simulink model "MPC_VS_FOCCopy_ST_Psim12"  (R2021a)
settings: Solver=VariableStepAuto  StartTime=0.0  StopTime=0.3  FixedStep=1/150000  MaxStep=1e-6
libraries: spsMosfetLib x12, simulink x7, pid_lib x3, spsFirstOrderFilterLib x2, spsPermanentMagnetSynchronousMachineLib x2, spsCurrentMeasurementLib x2, spsDCVoltageSourceLib x2, spsThreePhaseVIMeasurementLib x2, spsabctodq0Lib x2, spsSVPWMGenerator2LevelLib x1, spsdq0toAlphaBetaZeroLib x1, spspowerguiLib x1
settings Model: Creator=Hassan Alam  LastModifiedBy=zero
settings SolverCC: ZeroCrossAlgorithm=Adaptive
settings DebuggingCC: MaskedZcDiagnostic=none  IgnoredZcDiagnostic=none  SFMachineParentedDataDiag=warning  ArithmeticOperatorsInVariantConditions=warning
settings SFSimCC: CustomCodeUndefinedFunction=UseInterfaceOnly

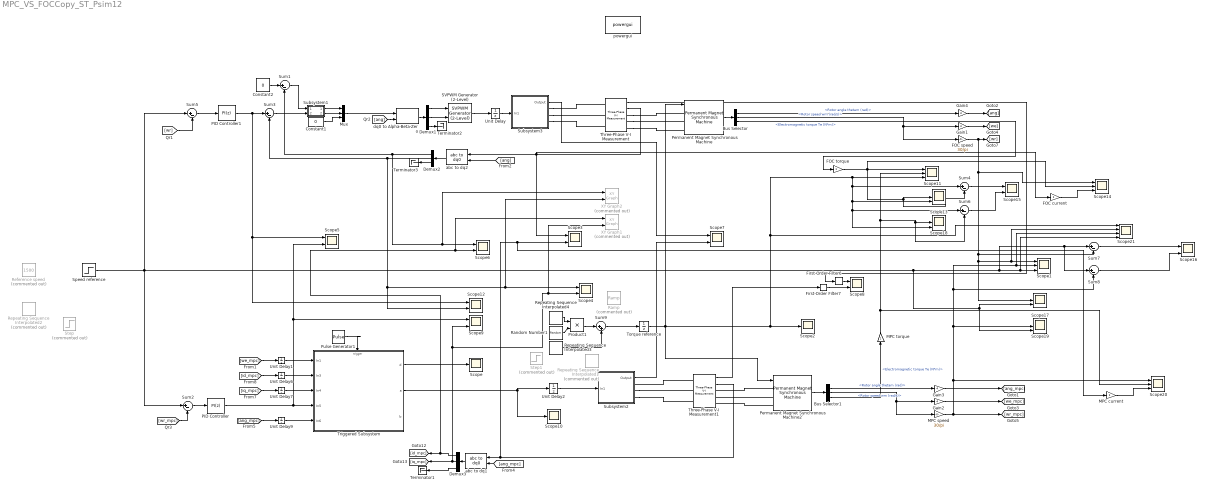
== system MPC_VS_FOCCopy_ST_Psim12 ==
  Bus Selector : BusSelector  OutputSignals=Rotor angle thetam (rad),Rotor speed wm (rad/s),Electromagnetic torque Te (N*m)
  Bus Selector1 : BusSelector  OutputSignals=Rotor angle thetam (rad),Rotor speed wm (rad/s),Electromagnetic torque Te (N*m)
  Constant1 : Constant  Value=0
  Constant2 : Constant  Value=0
  Demux1 : Demux  Outputs=3
  Demux2 : Demux  Outputs=3
  Demux3 : Demux  Outputs=3
  FOC current : Gain
  FOC speed : Gain  Gain=30/pi
  FOC torque : Gain
  First-Order Filter6 : spsFirstOrderFilterLib/First-Order Filter  FilterType=Lowpass  Tc=1e-3  Ts=0  Initialize=on  Vac_Init=[0, 0, 60]  Vdc_Init=0  PlotResponse=off  FreqRange="[0,  200,  1]"
  First-Order Filter7 : spsFirstOrderFilterLib/First-Order Filter  FilterType=Lowpass  Tc=1e-3  Ts=0  Initialize=on  Vac_Init=[0, 0, 60]  Vdc_Init=0  PlotResponse=off  FreqRange="[0,  200,  1]"
  Gain{1..4} (4 alike) : Gain  Gain=4
  MPC current : Gain
  MPC speed : Gain  Gain=30/pi
  MPC torque : Gain
  Mux : Mux  Inputs=3
  PID Controller : pid_lib/PID Controller  Controller=PI  Form=Parallel  TimeDomain=Discrete-time  UseExternalTs=off  SampleTime=1/4000  IntegratorMethod=Forward Euler  FilterMethod=Forward Euler  ControllerParametersSource=internal  P=0.02  I=20  D=0  UseFilter=on  N=100  TunerSelectOption=Transfer Function Based (PID Tuner App)  InitialConditionSource=internal  InitialConditionForIntegrator=0  InitialConditionForFilter=0  DifferentiatorICPrevScaledInput=0  ExternalReset=none  TrackingMode=off  Kt=1  LimitOutput=on  SatLimitsSource=internal  UpperSaturationLimit=3  LowerSaturationLimit=-3  LinearizeAsGain=on  AntiWindupMode=clamping  Kb=1  POutMin=[]  POutMax=[]  IOutMin=[]  IOutMax=[]  DOutMin=[]  DOutMax=[]  NOutMin=[]  NOutMax=[]  SumOutMin=[]  SumOutMax=[]  SaturationOutMin=[]  SaturationOutMax=[]  PParamMin=[]  PParamMax=[]  IParamMin=[]  IParamMax=[]  DParamMin=[]  DParamMax=[]  NParamMin=[]  NParamMax=[]  KbParamMin=[]  KbParamMax=[]  KtParamMin=[]  KtParamMax=[]  KbOutMin=[]  KbOutMax=[]  KtOutMin=[]  KtOutMax=[]  IntegratorOutMin=[]  IntegratorOutMax=[]  FilterOutMin=[]  FilterOutMax=[]  SumI1OutMin=[]  SumI1OutMax=[]  SumI2OutMin=[]  SumI2OutMax=[]  SumI3OutMin=[]  SumI3OutMax=[]  SumI4OutMin=[]  SumI4OutMax=[]  SumDOutMin=[]  SumDOutMax=[]  DifferentiatorOutMin=[]  DifferentiatorOutMax=[]  FilterDiffOutCoefMin=[]  FilterDiffOutCoefMax=[]  ReciprocalOutMin=[]  ReciprocalOutMax=[]  SumDenOutMin=[]  SumDenOutMax=[]  SumNumOutMin=[]  SumNumOutMax=[]  DivideOutMin=[]  DivideOutMax=[]  UdiffTsProdOutMin=[]  UdiffTsProdOutMax=[]  NTsProdOutMin=[]  NTsProdOutMax=[]  UintegralTsProdOutMin=[]  UintegralTsProdOutMax=[]  UngainTsProdOutMin=[]  UngainTsProdOutMax=[]  IntegratorContinuousStateAttributes=''  IntegratorStateMustResolveToSignalObject=off  IntegratorRTWStateStorageClass=Auto  FilterContinuousStateAttributes=''  FilterStateMustResolveToSignalObject=off  FilterRTWStateStorageClass=Auto  ParallelPVariant=InternalParameters  IdealPVariant=Disabled  IVariant=InternalParameters  DVariant=Disabled  IntegratorVariant=Discrete  SatVariant=Enabled  AWVariant=DiscClampingParallel  PCopyVariant=Disabled  TRVariant=Disabled  FdbkBlocksVariant=Forward  IdealPFdbkVariant=Disabled  SatFdbkVariant=Disabled  DerivativeFilterVariant=Disabled  NVariant=Disabled  NCopyVariant=Disabled_SignalSpec  FilterICVariant=Disabled  IntegratorICVariant=InternalICs  ExternalResetVariant=Disabled  TRSumVariant=Passthrough  SumFdbkVariant=Disabled  SumVariant=Sum_PI  TsampFilterVariant=InternalTs  TsampNgainVariant=Passthrough  TsampIntegralVariant=Passthrough  ExternalSaturationOutDataTypeStr=Inherit: Same as second input
  PID Controller1 : pid_lib/PID Controller  Controller=PI  Form=Parallel  TimeDomain=Discrete-time  UseExternalTs=off  SampleTime=1/4000  IntegratorMethod=Forward Euler  FilterMethod=Forward Euler  ControllerParametersSource=internal  P=0.02  I=20  D=0  UseFilter=on  N=100  TunerSelectOption=Transfer Function Based (PID Tuner App)  InitialConditionSource=internal  InitialConditionForIntegrator=0  InitialConditionForFilter=0  DifferentiatorICPrevScaledInput=0  ExternalReset=none  TrackingMode=off  Kt=1  LimitOutput=on  SatLimitsSource=internal  UpperSaturationLimit=3  LowerSaturationLimit=-3  LinearizeAsGain=on  AntiWindupMode=clamping  Kb=1  POutMin=[]  POutMax=[]  IOutMin=[]  IOutMax=[]  DOutMin=[]  DOutMax=[]  NOutMin=[]  NOutMax=[]  SumOutMin=[]  SumOutMax=[]  SaturationOutMin=[]  SaturationOutMax=[]  PParamMin=[]  PParamMax=[]  IParamMin=[]  IParamMax=[]  DParamMin=[]  DParamMax=[]  NParamMin=[]  NParamMax=[]  KbParamMin=[]  KbParamMax=[]  KtParamMin=[]  KtParamMax=[]  KbOutMin=[]  KbOutMax=[]  KtOutMin=[]  KtOutMax=[]  IntegratorOutMin=[]  IntegratorOutMax=[]  FilterOutMin=[]  FilterOutMax=[]  SumI1OutMin=[]  SumI1OutMax=[]  SumI2OutMin=[]  SumI2OutMax=[]  SumI3OutMin=[]  SumI3OutMax=[]  SumI4OutMin=[]  SumI4OutMax=[]  SumDOutMin=[]  SumDOutMax=[]  DifferentiatorOutMin=[]  DifferentiatorOutMax=[]  FilterDiffOutCoefMin=[]  FilterDiffOutCoefMax=[]  ReciprocalOutMin=[]  ReciprocalOutMax=[]  SumDenOutMin=[]  SumDenOutMax=[]  SumNumOutMin=[]  SumNumOutMax=[]  DivideOutMin=[]  DivideOutMax=[]  UdiffTsProdOutMin=[]  UdiffTsProdOutMax=[]  NTsProdOutMin=[]  NTsProdOutMax=[]  UintegralTsProdOutMin=[]  UintegralTsProdOutMax=[]  UngainTsProdOutMin=[]  UngainTsProdOutMax=[]  IntegratorContinuousStateAttributes=''  IntegratorStateMustResolveToSignalObject=off  IntegratorRTWStateStorageClass=Auto  FilterContinuousStateAttributes=''  FilterStateMustResolveToSignalObject=off  FilterRTWStateStorageClass=Auto  ParallelPVariant=InternalParameters  IdealPVariant=Disabled  IVariant=InternalParameters  DVariant=Disabled  IntegratorVariant=Discrete  SatVariant=Enabled  AWVariant=DiscClampingParallel  PCopyVariant=Disabled  TRVariant=Disabled  FdbkBlocksVariant=Forward  IdealPFdbkVariant=Disabled  SatFdbkVariant=Disabled  DerivativeFilterVariant=Disabled  NVariant=Disabled  NCopyVariant=Disabled_SignalSpec  FilterICVariant=Disabled  IntegratorICVariant=InternalICs  ExternalResetVariant=Disabled  TRSumVariant=Passthrough  SumFdbkVariant=Disabled  SumVariant=Sum_PI  TsampFilterVariant=InternalTs  TsampNgainVariant=Passthrough  TsampIntegralVariant=Passthrough  ExternalSaturationOutDataTypeStr=Inherit: Same as second input
  Permanent Magnet Synchronous Machine : spsPermanentMagnetSynchronousMachineLib/Permanent Magnet Synchronous Machine  NbPhases=3  FluxDistribution=Sinusoidal  RotorType=Round  MechanicalLoad=Torque Tm  PresetModel=No  ShowDetailedParameters=on  MeasurementBus=off  Resistance=0.75  Inductance=8.5e-3  dqInductances=[8.5e-3,8.5e-3]  La=0.0004  MachineConstant=Flux linkage established by magnets (V.s)  Flux=0.00666  VoltageCst=4.832  TorqueCst=0.03996  Flat=120  Mechanical=[2.66e-6 1.33e-6 4 0]  PolePairs=4  InitialConditions=[0,0, 0,0]  InitialConditions5ph=[0 0 0 0 0 0]  RefAngle=90 degrees behind phase A axis (modified Park)  IterativeDiscreteModel=Trapezoidal non iterative  TsBlock=-1  TsPowergui=0
  Permanent Magnet Synchronous Machine2 : spsPermanentMagnetSynchronousMachineLib/Permanent Magnet Synchronous Machine  NbPhases=3  FluxDistribution=Sinusoidal  RotorType=Round  MechanicalLoad=Torque Tm  PresetModel=No  ShowDetailedParameters=on  MeasurementBus=off  Resistance=0.75  Inductance=8.5e-3  dqInductances=[8.5e-3,8.5e-3]  La=0.0004  MachineConstant=Flux linkage established by magnets (V.s)  Flux=0.00666  VoltageCst=4.832  TorqueCst=0.03996  Flat=120  Mechanical=[2.66e-6 1.33e-6 4 0]  PolePairs=4  InitialConditions=[0,0, 0,0]  InitialConditions5ph=[0 0 0 0 0 0]  RefAngle=90 degrees behind phase A axis (modified Park)  IterativeDiscreteModel=Trapezoidal non iterative  TsBlock=-1  TsPowergui=0
  Product1 : Product
  Pulse Generator1 : DiscretePulseGenerator  PulseType=Time based  Period=1/40000  PulseWidth=5
  Ramp : simulink/Sources/Ramp  Commented=on  slope=1  start=0  InitialOutput=0
  Random Number1 : RandomNumber  Seed=123  SampleTime=1e-4*2
  Reference speed : Constant  Commented=on  Value=1500
  Repeating Sequence Interpolated1 : simulink/Sources/Repeating Sequence Interpolated  Commented=on  OutValues=[0 0 0.1 0.1 -0.1 -0.1].'  TimeValues=[0 0.1 0.10001 0.3 0.30001 0.4].'  LookUpMeth=Interpolation-Use End Values  tsamp=1e-6  OutMin=[]  OutMax=[]  OutDataTypeStr=double  OutputDataTypeScalingMode=double  OutDataType=fixdt(0,8)  OutScaling=2^-10
  Repeating Sequence Interpolated2 : simulink/Sources/Repeating Sequence Interpolated  Commented=on  OutValues=[1500 1500 800 800 1200 1200 500 500 1000 1000 1500 1500 0].'  TimeValues=[0 0.0229 0.023 0.0499 0.05 0.095 0.10 0.159 0.16 0.20 0.22 0.27 0.3].'/0.333  LookUpMeth=Interpolation-Use End Values  tsamp=1e-6  OutMin=[]  OutMax=[]  OutDataTypeStr=double  OutputDataTypeScalingMode=double  OutDataType=fixdt(0,8)  OutScaling=2^-10
  Repeating Sequence Interpolated3 : simulink/Sources/Repeating Sequence Interpolated  OutValues=[0 0.05 0.1 0.1 0.1 0.125 0.125 0.05 0].'*0.7  TimeValues=[0 0.01 0.02 0.05 0.15 0.16 0.25 0.27 0.3].'  LookUpMeth=Interpolation-Use End Values  tsamp=1e-6  OutMin=[]  OutMax=[]  OutDataTypeStr=double  OutputDataTypeScalingMode=double  OutDataType=fixdt(0,8)  OutScaling=2^-10
  Repeating Sequence Interpolated4 : simulink/Sources/Repeating Sequence Interpolated  OutValues=[0 0.008 0.015 0.015 0.015 0.02 0.02 0.008 0].'  TimeValues=[0 0.01 0.02 0.05 0.15 0.16 0.25 0.27 0.3].'  LookUpMeth=Interpolation-Use End Values  tsamp=1e-6  OutMin=[]  OutMax=[]  OutDataTypeStr=double  OutputDataTypeScalingMode=double  OutDataType=fixdt(0,8)  OutScaling=2^-10
  SVPWM Generator (2-Level) : spsSVPWMGenerator2LevelLib/SVPWM Generator (2-Level)  InputType=alpha-beta components  SwitchingPattern=Pattern #1  Fc=40000  ParUref=[0.8 -30 50]  Ts=0
      settings: SourceProductBaseCode=PS
  Scope : Scope
  Scope{1,11,13..14,17..20} (8 alike) : Scope  NumInputPorts=3
  Scope10 : Scope
  Scope{3..9,12,15..16} (10 alike) : Scope  NumInputPorts=2
  Scope2 : Scope
  Scope21 : Scope  NumInputPorts=4
  Speed reference : Step  Time=0.2  Before=1500  After=1500  SampleTime=0
  Step : Step  Commented=on  Time=0  After=800  SampleTime=0
  Step1 : Step  Commented=on  Time=0.1  After=0.1  SampleTime=0
  Subsystem1 : Subsystem
  Subsystem2 : Subsystem
  Subsystem3 : Subsystem
  Sum{1..8} (8 alike) : Sum  Inputs=|+-
  Sum9 : Sum  Inputs=|++
  Terminator1 : Terminator
  Terminator2 : Terminator
  Terminator3 : Terminator
  Three-Phase V-I Measurement : spsThreePhaseVIMeasurementLib/Three-Phase V-I Measurement  VoltageMeasurement=phase-to-phase  SetLabelV=off  LabelV=Vabc  Vpu=off  VpuLL=off  CurrentMeasurement=yes  SetLabelI=off  LabelI=Iabc  Ipu=off  Pbase=100e6  Vbase=500e3  OutputType=Complex  PhasorSimulation=off  PSBequivalent=0
  Three-Phase V-I Measurement1 : spsThreePhaseVIMeasurementLib/Three-Phase V-I Measurement  VoltageMeasurement=phase-to-phase  SetLabelV=off  LabelV=Vabc  Vpu=off  VpuLL=off  CurrentMeasurement=yes  SetLabelI=off  LabelI=Iabc  Ipu=off  Pbase=100e6  Vbase=500e3  OutputType=Complex  PhasorSimulation=off  PSBequivalent=0
  Torque reference : UnitDelay  SampleTime=1e-6  HasFrameUpgradeWarning=on
  Triggered Subsystem : Subsystem  TreatAsAtomicUnit=on
  Unit Delay : UnitDelay  SampleTime=1e-6  HasFrameUpgradeWarning=on
  Unit Delay{1,6..7,9} (4 alike) : UnitDelay  SampleTime=-1  HasFrameUpgradeWarning=on
  Unit Delay2 : UnitDelay  SampleTime=1e-6  HasFrameUpgradeWarning=on
  XY Graph1 : simulink/Sinks/XY Graph  Commented=on  xmin=-5  xmax=5  ymin=-5  ymax=5  st=-1
  XY Graph2 : simulink/Sinks/XY Graph  Commented=on  xmin=-5  xmax=5  ymin=-5  ymax=5  st=-1
  abc to dq1 : spsabctodq0Lib/abc to dq0  Alignment=90 degrees behind phase A axis
  abc to dq2 : spsabctodq0Lib/abc to dq0  Alignment=90 degrees behind phase A axis
  dq0 to Alpha-Beta-Zero : spsdq0toAlphaBetaZeroLib/dq0 to Alpha-Beta-Zero  Alignment=90 degrees behind phase A axis
      settings: SourceProductBaseCode=PS
  powergui : spspowerguiLib/powergui  Priority=1  SimulationMode=Continuous  SampleTime=1e-6  frequency=60  Iterations=50  frequencyindice=0  Pbase=100e6  ErrMax=1e-4  UnitsV=kV  UnitsW=MW  buscounter=0  FunctionMessages=off  echomessages=off  EnableUseOfTLC=off  CurrentSourceSwitches=off  DisableSnubberDevices=off  DisableRonSwitches=off  DisableVfSwitches=off  DisplayEquations=off  AutomaticDiscreteSolvers=off  SolverType=Tustin/Backward Euler (TBE)  Interpol=off  ExternalGateDelay=off  methode=off  Ts=100  x0status=blocks  SPID=on  SwTol=0  HookPort=off  NonlinearTolerance=1e-4  nMaxIteration=100  ContinueOnMaxIteration=off  RestoreLinks=warning  ResistiveCurrentMeasurement=off  Frange=[0:2:500]  Ylog=off  Xlog=on  ShowGrid=off  save=off  variable=ZData  structure=0  ZoomFFT=off  StartTime=0.0  cycles=1  DisplayStyle=1  fundamental=60  FreqAxis=off  MaxFrequency=1000  frequencyindicesteady=1  RmsSteady=1  display=off
  wires:
  [wr] -> Sum5/2
  Unit Delay7/1 -> Triggered Subsystem/3(In4)
  [we_mpc] -> Unit Delay1/1
  [ang_mpc] -> Unit Delay9/1
  [iq_mpc] -> Unit Delay7/1
  PID Controller/1 -> Scope9/1, Scope5/2, Triggered Subsystem/4(In5)
  Unit Delay1/1 -> Triggered Subsystem/1(In1)
  [id_mpc] -> Unit Delay6/1
  Unit Delay6/1 -> Triggered Subsystem/2(In3)
  Unit Delay9/1 -> Triggered Subsystem/5(In6)
  Pulse Generator1/1 -> Triggered Subsystem/Trigger
  Constant2/1 -> Sum1/1
  dq0 to Alpha-Beta-Zero/1 -> Demux1/1
  Demux1/2 -> SVPWM Generator (2-Level)/2
  Demux1/1 -> SVPWM Generator (2-Level)/1
  Demux1/3 -> Terminator2/1
  [ang] -> dq0 to Alpha-Beta-Zero/2
  Constant1/1 -> Mux/3
  abc to dq2/1 -> Demux2/1
  Gain4/1 -> [ang]
  Gain1/1 -> [we]
  [ang] -> abc to dq2/2
  Demux2/3 -> Terminator3/1
  Demux3/3 -> Terminator1/1
  [ang_mpc] -> abc to dq1/2
  abc to dq1/1 -> Demux3/1
  Three-Phase V-I Measurement1/2 -> MPC current/1, Scope3/2, abc to dq1/1
  Three-Phase V-I Measurement/2 -> Scope3/1, FOC current/1, abc to dq2/1
  Demux2/2 -> Sum3/2, Scope12/2, XY Graph2/2, Scope4/1
  Demux3/2 -> [iq_mpc], Scope9/2, XY Graph1/2, Scope4/2
  Demux3/1 -> XY Graph1/1, Scope6/2, [id_mpc]
  Demux2/1 -> XY Graph2/1, Scope6/1, Sum1/2
  First-Order Filter7/1 -> Scope8/2
  First-Order Filter6/1 -> Scope8/1
  Three-Phase V-I Measurement1/1 -> First-Order Filter7/1
  Three-Phase V-I Measurement/1 -> First-Order Filter6/1
  Sum5/1 -> PID Controller1/1
  Speed reference/1 -> Sum5/1, Scope19/3, Scope17/3, Sum8/1, Sum7/1, Scope21/4, Scope1/3, Sum2/1
  [wr_mpc] -> Sum2/2
  Sum1/1 -> Subsystem1/1(In1)
  Sum3/1 -> Subsystem1/2(In2)
  Subsystem1/1(Out1) -> Mux/1
  Subsystem1/2(Out2) -> Mux/2
  Sum2/1 -> PID Controller/1
  Torque reference/1 -> Scope21/1, Sum4/1, Scope13/3, Scope18/3, Sum6/1, Scope11/3, Scope2/1, Permanent Magnet Synchronous Machine2/1, Permanent Magnet Synchronous Machine/1
  Subsystem3/1(Output) -> Scope7/1
  PID Controller1/1 -> Scope12/1, Scope5/1, Sum3/1
  Mux/1 -> dq0 to Alpha-Beta-Zero/1
  SVPWM Generator (2-Level)/1 -> Unit Delay/1
  Unit Delay/1 -> Subsystem3/1(In1)
  Permanent Magnet Synchronous Machine/1 -> Bus Selector/1
  Bus Selector/1 -> Gain4/1  "<Rotor angle thetam (rad)>"
  Bus Selector/2 -> FOC speed/1, Gain1/1  "<Rotor speed wm (rad/s)>"
  Bus Selector1/2 -> Gain2/1, MPC speed/1  "<Rotor speed wm (rad/s)>"
  Bus Selector1/1 -> Gain3/1  "<Rotor angle thetam (rad)>"
  Permanent Magnet Synchronous Machine2/1 -> Bus Selector1/1
  Gain2/1 -> [we_mpc]
  Gain3/1 -> [ang_mpc]
  Unit Delay2/1 -> Subsystem2/1(In1)
  Subsystem2/1(Output) -> Scope7/2
  Bus Selector/3 -> FOC torque/1  "<Electromagnetic torque Te (N*m)>"
  Bus Selector1/3 -> MPC torque/1  "<Electromagnetic torque Te (N*m)>"
  MPC torque/1 -> Scope20/2, Scope18/2, Sum6/2, Scope11/2
  FOC torque/1 -> Scope14/2, Sum4/2, Scope13/2, Scope11/1
  Sum6/1 -> Scope15/2
  Sum4/1 -> Scope15/1
  Sum7/1 -> Scope16/1
  Sum8/1 -> Scope16/2
  FOC speed/1 -> Scope14/1, Scope17/2, Scope21/2, Scope1/1, Sum7/2, [wr]
  MPC speed/1 -> Scope19/2, Sum8/2, Scope21/3, Scope1/2, Scope20/1, [wr_mpc]
  Random Number1/1 -> Product1/2
  Repeating Sequence Interpolated4/1 -> Product1/1
  Repeating Sequence Interpolated3/1 -> Sum9/2
  Product1/1 -> Sum9/1
  Triggered Subsystem/2(a) -> Scope10/1, Unit Delay2/1
  Triggered Subsystem/1(d) -> Scope/1
  FOC current/1 -> Scope14/3
  MPC current/1 -> Scope20/3
  Sum9/1 -> Torque reference/1
  connections:
  Subsystem3/RConn1 -- Three-Phase V-I Measurement/LConn1
  Subsystem3/RConn2 -- Three-Phase V-I Measurement/LConn2
  Subsystem3/RConn3 -- Three-Phase V-I Measurement/LConn3
  Three-Phase V-I Measurement/RConn1 -- Permanent Magnet Synchronous Machine/LConn1
  Three-Phase V-I Measurement/RConn2 -- Permanent Magnet Synchronous Machine/LConn2
  Three-Phase V-I Measurement/RConn3 -- Permanent Magnet Synchronous Machine/LConn3
  Permanent Magnet Synchronous Machine2/LConn3 -- Three-Phase V-I Measurement1/RConn3
  Permanent Magnet Synchronous Machine2/LConn1 -- Three-Phase V-I Measurement1/RConn1
  Subsystem2/RConn2 -- Three-Phase V-I Measurement1/LConn2
  Subsystem2/RConn3 -- Three-Phase V-I Measurement1/LConn3
  Three-Phase V-I Measurement1/LConn1 -- Subsystem2/RConn1
  Permanent Magnet Synchronous Machine2/LConn2 -- Three-Phase V-I Measurement1/RConn2

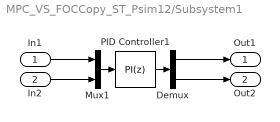
== system MPC_VS_FOCCopy_ST_Psim12/Subsystem1 ==
  In1 : Inport
  In2 : Inport  Port=2
  Demux : Demux  Outputs=2
  Mux1 : Mux  Inputs=2
  PID Controller1 : pid_lib/PID Controller  Controller=PI  Form=Parallel  TimeDomain=Discrete-time  UseExternalTs=off  SampleTime=1/40000  IntegratorMethod=Forward Euler  FilterMethod=Forward Euler  ControllerParametersSource=internal  P=1  I=800  D=0  UseFilter=on  N=100  TunerSelectOption=Transfer Function Based (PID Tuner App)  InitialConditionSource=internal  InitialConditionForIntegrator=0  InitialConditionForFilter=0  DifferentiatorICPrevScaledInput=0  ExternalReset=none  TrackingMode=off  Kt=1  LimitOutput=off  SatLimitsSource=internal  UpperSaturationLimit=3  LowerSaturationLimit=-3  LinearizeAsGain=on  AntiWindupMode=clamping  Kb=1  POutMin=[]  POutMax=[]  IOutMin=[]  IOutMax=[]  DOutMin=[]  DOutMax=[]  NOutMin=[]  NOutMax=[]  SumOutMin=[]  SumOutMax=[]  SaturationOutMin=[]  SaturationOutMax=[]  PParamMin=[]  PParamMax=[]  IParamMin=[]  IParamMax=[]  DParamMin=[]  DParamMax=[]  NParamMin=[]  NParamMax=[]  KbParamMin=[]  KbParamMax=[]  KtParamMin=[]  KtParamMax=[]  KbOutMin=[]  KbOutMax=[]  KtOutMin=[]  KtOutMax=[]  IntegratorOutMin=[]  IntegratorOutMax=[]  FilterOutMin=[]  FilterOutMax=[]  SumI1OutMin=[]  SumI1OutMax=[]  SumI2OutMin=[]  SumI2OutMax=[]  SumI3OutMin=[]  SumI3OutMax=[]  SumI4OutMin=[]  SumI4OutMax=[]  SumDOutMin=[]  SumDOutMax=[]  DifferentiatorOutMin=[]  DifferentiatorOutMax=[]  FilterDiffOutCoefMin=[]  FilterDiffOutCoefMax=[]  ReciprocalOutMin=[]  ReciprocalOutMax=[]  SumDenOutMin=[]  SumDenOutMax=[]  SumNumOutMin=[]  SumNumOutMax=[]  DivideOutMin=[]  DivideOutMax=[]  UdiffTsProdOutMin=[]  UdiffTsProdOutMax=[]  NTsProdOutMin=[]  NTsProdOutMax=[]  UintegralTsProdOutMin=[]  UintegralTsProdOutMax=[]  UngainTsProdOutMin=[]  UngainTsProdOutMax=[]  IntegratorContinuousStateAttributes=''  IntegratorStateMustResolveToSignalObject=off  IntegratorRTWStateStorageClass=Auto  FilterContinuousStateAttributes=''  FilterStateMustResolveToSignalObject=off  FilterRTWStateStorageClass=Auto  ParallelPVariant=InternalParameters  IdealPVariant=Disabled  IVariant=InternalParameters  DVariant=Disabled  IntegratorVariant=Discrete  SatVariant=Disabled  AWVariant=Passthrough  PCopyVariant=Disabled  TRVariant=Disabled  FdbkBlocksVariant=Forward  IdealPFdbkVariant=Disabled  SatFdbkVariant=Disabled  DerivativeFilterVariant=Disabled  NVariant=Disabled  NCopyVariant=Disabled_SignalSpec  FilterICVariant=Disabled  IntegratorICVariant=InternalICs  ExternalResetVariant=Disabled  TRSumVariant=Passthrough  SumFdbkVariant=Disabled  SumVariant=Sum_PI  TsampFilterVariant=InternalTs  TsampNgainVariant=Passthrough  TsampIntegralVariant=Passthrough  ExternalSaturationOutDataTypeStr=Inherit: Same as second input
  Out1 : Outport
  Out2 : Outport  Port=2
  wires:
  In1/1 -> Mux1/1
  Mux1/1 -> PID Controller1/1
  Demux/2 -> Out2/1
  PID Controller1/1 -> Demux/1
  Demux/1 -> Out1/1
  In2/1 -> Mux1/2

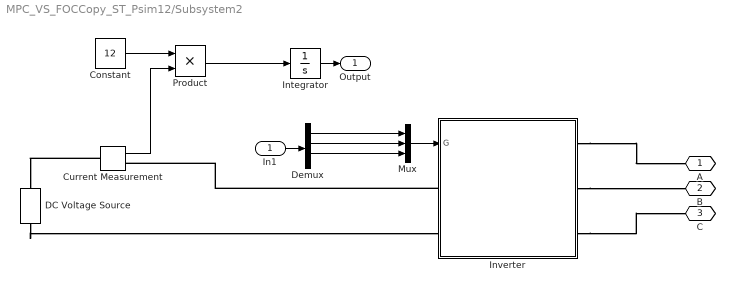
== system MPC_VS_FOCCopy_ST_Psim12/Subsystem2 ==
  In1 : Inport
  Constant : Constant  Value=12
  Current Measurement : spsCurrentMeasurementLib/Current Measurement  PhasorSimulation=off  OutputType=Complex  PSBequivalent=0
  DC Voltage Source : spsDCVoltageSourceLib/DC Voltage Source  Amplitude=12  Measurements=None
  Demux : Demux  Outputs=6
  Integrator : Integrator
  Inverter : Subsystem
  Mux : Mux  Inputs=3
  Product : Product
  A : PMIOPort  Side=Right
  B : PMIOPort  Port=2  Side=Right
  C : PMIOPort  Port=3  Side=Right
  Output : Outport
  wires:
  Current Measurement/1 -> Product/2
  Integrator/1 -> Output/1
  Constant/1 -> Product/1
  Product/1 -> Integrator/1
  Demux/5 -> Mux/3
  Mux/1 -> Inverter/1(G)
  Demux/1 -> Mux/1
  Demux/3 -> Mux/2
  In1/1 -> Demux/1
  connections:
  Inverter/LConn1 -- Current Measurement/RConn1
  DC Voltage Source/LConn1 -- Inverter/LConn2
  Current Measurement/LConn1 -- DC Voltage Source/RConn1
  Inverter/RConn1 -- A/RConn1
  Inverter/RConn2 -- B/RConn1
  Inverter/RConn3 -- C/RConn1

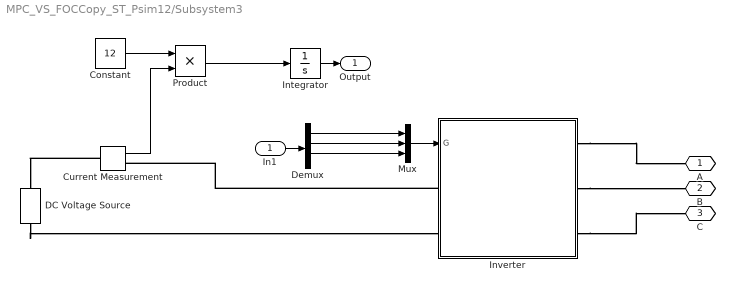
== system MPC_VS_FOCCopy_ST_Psim12/Subsystem3 ==
  In1 : Inport
  Constant : Constant  Value=12
  Current Measurement : spsCurrentMeasurementLib/Current Measurement  PhasorSimulation=off  OutputType=Complex  PSBequivalent=0
  DC Voltage Source : spsDCVoltageSourceLib/DC Voltage Source  Amplitude=12  Measurements=None
  Demux : Demux  Outputs=6
  Integrator : Integrator
  Inverter : Subsystem
  Mux : Mux  Inputs=3
  Product : Product
  A : PMIOPort  Side=Right
  B : PMIOPort  Port=2  Side=Right
  C : PMIOPort  Port=3  Side=Right
  Output : Outport
  wires:
  In1/1 -> Demux/1
  Demux/3 -> Mux/2
  Demux/1 -> Mux/1
  Mux/1 -> Inverter/1(G)
  Demux/5 -> Mux/3
  Product/1 -> Integrator/1
  Constant/1 -> Product/1
  Integrator/1 -> Output/1
  Current Measurement/1 -> Product/2
  connections:
  Inverter/RConn3 -- C/RConn1
  Inverter/RConn2 -- B/RConn1
  Inverter/RConn1 -- A/RConn1
  Current Measurement/LConn1 -- DC Voltage Source/RConn1
  DC Voltage Source/LConn1 -- Inverter/LConn2
  Inverter/LConn1 -- Current Measurement/RConn1

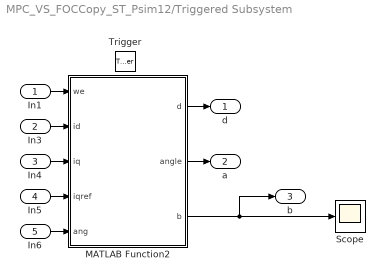
== system MPC_VS_FOCCopy_ST_Psim12/Triggered Subsystem ==
  In1 : Inport
  In3 : Inport  Port=2
  In4 : Inport  Port=3
  In5 : Inport  Port=4
  In6 : Inport  Port=5
  Trigger : TriggerPort  VariantControl=Variant
  MATLAB Function2 : MATLAB Function  TreatAsAtomicUnit=on
  Scope : Scope
  d : Outport  VectorParamsAs1DForOutWhenUnconnected=off
  a : Outport  Port=2  VectorParamsAs1DForOutWhenUnconnected=off
  b : Outport  Port=3  VectorParamsAs1DForOutWhenUnconnected=off
  wires:
  In1/1 -> MATLAB Function2/1(we)
  In3/1 -> MATLAB Function2/2(id)
  In4/1 -> MATLAB Function2/3(iq)
  In5/1 -> MATLAB Function2/4(iqref)
  In6/1 -> MATLAB Function2/5(ang)
  MATLAB Function2/1(d) -> d/1
  MATLAB Function2/2(angle) -> a/1
  MATLAB Function2/3(b) -> b/1, Scope/1

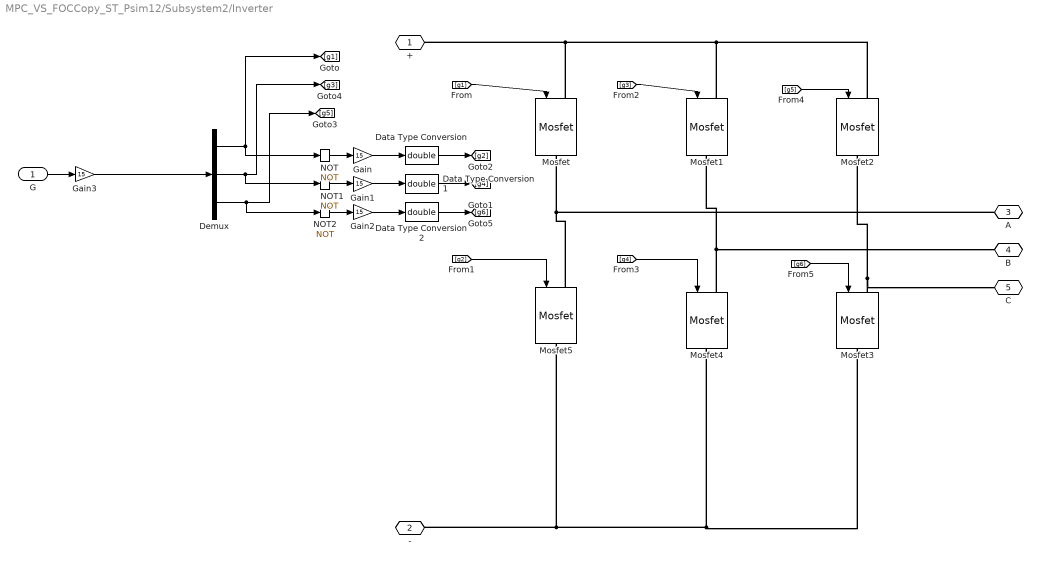
== system MPC_VS_FOCCopy_ST_Psim12/Subsystem2/Inverter ==
  G : Inport
  Data Type Conversion : DataTypeConversion  OutDataTypeStr=double
  Data Type Conversion1 : DataTypeConversion  OutDataTypeStr=double
  Data Type Conversion2 : DataTypeConversion  OutDataTypeStr=double
  Demux : Demux  Outputs=3
  Gain{,1..3} (4 alike) : Gain  Gain=15
  Mosfet{,1..5} (6 alike) : spsMosfetLib/Mosfet  Ron=0.052  Lon=0  Rd=0.052  Vfd=0.8  IC=0  Rs=1e5  Cs=inf  Measurements=off
  NOT : Logic  Operator=NOT  IconShape=distinctive  AllPortsSameDT=off  OutDataTypeStr=boolean
  NOT1 : Logic  Operator=NOT  IconShape=distinctive  AllPortsSameDT=off  OutDataTypeStr=boolean
  NOT2 : Logic  Operator=NOT  IconShape=distinctive  AllPortsSameDT=off  OutDataTypeStr=boolean
  + : PMIOPort  Side=Left
  - : PMIOPort  Port=2  Side=Left
  A : PMIOPort  Port=3  Side=Right
  B : PMIOPort  Port=4  Side=Right
  C : PMIOPort  Port=5  Side=Right
  wires:
  [g2] -> Mosfet5/1
  [g6] -> Mosfet3/1
  [g1] -> Mosfet/1
  G/1 -> Gain3/1
  [g3] -> Mosfet1/1
  [g4] -> Mosfet4/1
  Demux/2 -> NOT1/1, [g3]
  Demux/3 -> NOT2/1, [g5]
  NOT/1 -> Gain/1
  NOT1/1 -> Gain1/1
  NOT2/1 -> Gain2/1
  Gain/1 -> Data Type Conversion/1
  Gain1/1 -> Data Type Conversion1/1
  Gain2/1 -> Data Type Conversion2/1
  Data Type Conversion/1 -> [g2]
  Data Type Conversion1/1 -> [g4]
  Data Type Conversion2/1 -> [g6]
  [g5] -> Mosfet2/1
  Gain3/1 -> Demux/1
  Demux/1 -> [g1], NOT/1
  connections:
  Mosfet/RConn1 -- Mosfet5/LConn1 -- A/RConn1
  Mosfet1/RConn1 -- B/RConn1 -- Mosfet4/LConn1
  Mosfet2/RConn1 -- C/RConn1 -- Mosfet3/LConn1
  Mosfet1/LConn1 -- Mosfet2/LConn1 -- Mosfet/LConn1 -- +/RConn1
  -/RConn1 -- Mosfet5/RConn1 -- Mosfet3/RConn1 -- Mosfet4/RConn1

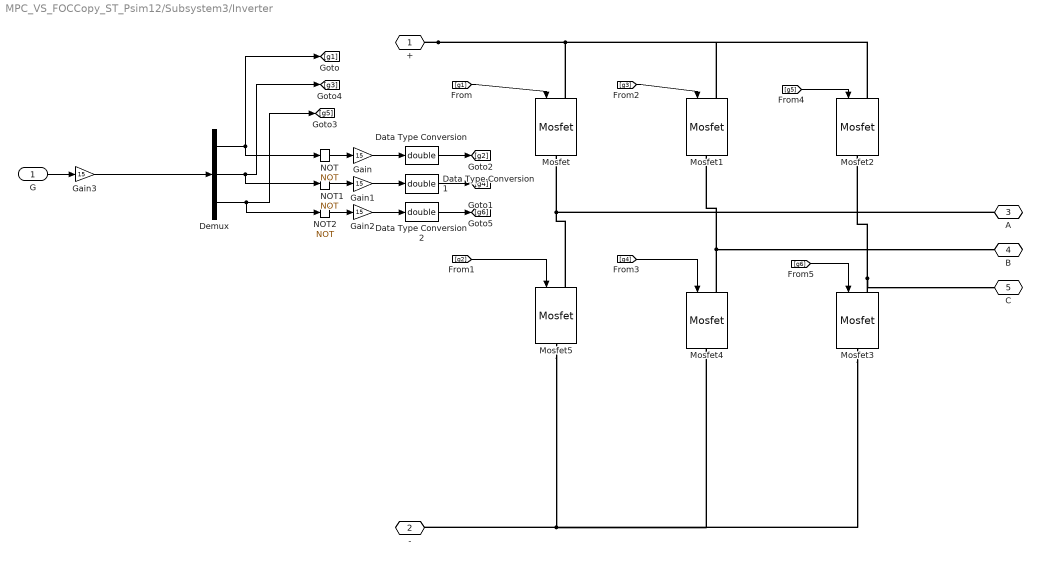
== system MPC_VS_FOCCopy_ST_Psim12/Subsystem3/Inverter ==
  G : Inport
  Data Type Conversion : DataTypeConversion  OutDataTypeStr=double
  Data Type Conversion1 : DataTypeConversion  OutDataTypeStr=double
  Data Type Conversion2 : DataTypeConversion  OutDataTypeStr=double
  Demux : Demux  Outputs=3
  Gain{,1..3} (4 alike) : Gain  Gain=15
  Mosfet{,1..5} (6 alike) : spsMosfetLib/Mosfet  Ron=0.052  Lon=0  Rd=0.052  Vfd=0.8  IC=0  Rs=1e5  Cs=inf  Measurements=off
  NOT : Logic  Operator=NOT  IconShape=distinctive  AllPortsSameDT=off  OutDataTypeStr=boolean
  NOT1 : Logic  Operator=NOT  IconShape=distinctive  AllPortsSameDT=off  OutDataTypeStr=boolean
  NOT2 : Logic  Operator=NOT  IconShape=distinctive  AllPortsSameDT=off  OutDataTypeStr=boolean
  + : PMIOPort  Side=Left
  - : PMIOPort  Port=2  Side=Left
  A : PMIOPort  Port=3  Side=Right
  B : PMIOPort  Port=4  Side=Right
  C : PMIOPort  Port=5  Side=Right
  wires:
  Demux/1 -> NOT/1, [g1]
  Gain3/1 -> Demux/1
  [g5] -> Mosfet2/1
  Data Type Conversion2/1 -> [g6]
  Data Type Conversion1/1 -> [g4]
  Data Type Conversion/1 -> [g2]
  Gain2/1 -> Data Type Conversion2/1
  Gain1/1 -> Data Type Conversion1/1
  Gain/1 -> Data Type Conversion/1
  NOT2/1 -> Gain2/1
  NOT1/1 -> Gain1/1
  NOT/1 -> Gain/1
  Demux/3 -> [g5], NOT2/1
  Demux/2 -> [g3], NOT1/1
  [g4] -> Mosfet4/1
  [g3] -> Mosfet1/1
  G/1 -> Gain3/1
  [g1] -> Mosfet/1
  [g6] -> Mosfet3/1
  [g2] -> Mosfet5/1
  connections:
  Mosfet3/RConn1 -- Mosfet4/RConn1 -- Mosfet5/RConn1 -- -/RConn1
  +/RConn1 -- Mosfet/LConn1 -- Mosfet2/LConn1 -- Mosfet1/LConn1
  Mosfet3/LConn1 -- C/RConn1 -- Mosfet2/RConn1
  Mosfet4/LConn1 -- B/RConn1 -- Mosfet1/RConn1
  A/RConn1 -- Mosfet5/LConn1 -- Mosfet/RConn1

== matlab function MPC_VS_FOCCopy_ST_Psim12/Triggered Subsystem/MATLAB Function2 ==
  data: we input; id input; iq input; iqref input; ang input; d output; angle output; b output
function [d,angle,b]  = MPC(we,id,iq,iqref,ang)

persistent oldState c;

if isempty(oldState)
    oldState = 1;
    psiq = 0;
    c  = 1;
end
b = 0;
Ts = 1/40000;
Vdc = 12;
L = 2*0.0004;
R = 2*0.75 + 2*0.052;
psiPM = 0.00666;

p = 0.5;
q = 0.5;
r = 0.25;
s = 0.0;

states = [1 0    0 1    0 1;
         1 0    1 0    0 1;
         0 1    1 0    0 1;
         0 1    1 0    1 0;
         0 1    0 1    1 0;
         1 0    0 1    1 0;
         0 1    0 1    0 1;
         1 0    1 0    1 0];

y = states(1,:)';
cost = [];

for i=1:length(states)
    Sa=states(i,1);
    Sb=states(i,3);
    Sc=states(i,5);
    
    Va=(Vdc*(2*Sa-Sb-Sc))/3;
    Vb=(Vdc*(2*Sb-Sa-Sc))/3;
    Vc=(Vdc*(2*Sc-Sb-Sa))/3;
    
    vsd = (2/3)*[sin(ang) sin(ang - (2*pi/3)) sin(ang + (2*pi/3))]*[Va Vb Vc]';
    vsq = (2/3)*[cos(ang) cos(ang - (2*pi/3)) cos(ang + (2*pi/3))]*[Va Vb Vc]';

    
    m = ~(states(i,:) == states(oldState,:));
    
    id_p = id;
    iq_p = iq;
    
    cTemp = 0;
    for x = 1:3
        xx = ((1-(R*Ts/L))*id_p)+(Ts*we*iq_p)+(vsd*Ts/L);
        yy = ((1-(R*Ts/L))*iq_p)-(Ts*we*id_p)-(psiPM*we*Ts/L)+(vsq*Ts/L);
    
        id_p = xx;
        iq_p = yy;
        
        ia = cos(ang)*id_p - sin(ang)*iq_p;
        ib = cos(ang - (2*pi/3))*id_p - sin(ang - (2*pi/3))*iq_p;
        ic = cos(ang + (2*pi/3))*id_p - sin(ang + (2*pi/3))*iq_p;

        if abs(iq_p) > 3
            cTemp = cTemp + 1000*abs(3 - sqrt(id_p^2 + iq_p^2));
        end
        
        mosfetLoss = 0;
        cTemp = cTemp + (0 - id_p)^2 + 1.8*(iqref - iq_p)^2;
    end
    

    cost = [cost  cTemp];
end

a = find(cost == min(cost));
a = a(end);
% if(abs(cost(a) - cost(oldState)) < 0.1)
%    a = oldState;
% end


if(a ~= oldState)
    c = c+1;
    
    if(a == 7 || a == 8)
       if(oldState == 1 || oldState == 3 || oldState == 5 || oldState == 8)
          a = 8; 
       elseif(oldState == 2 || oldState == 4 || oldState == 6 || oldState == 7)
           a = 7;
       end
    end
    
    oldState = a;
end
d=c;

b = a;

% angle = (a-1)*pi/3;
angle = states(a,:);
